simulink model "lab2sim"  (R2020a)
settings: Solver=VariableStepAuto  StartTime=0.0  StopTime=60  RelTol=1e-6
settings Model: Creator=ariana  LastModifiedBy=ariana

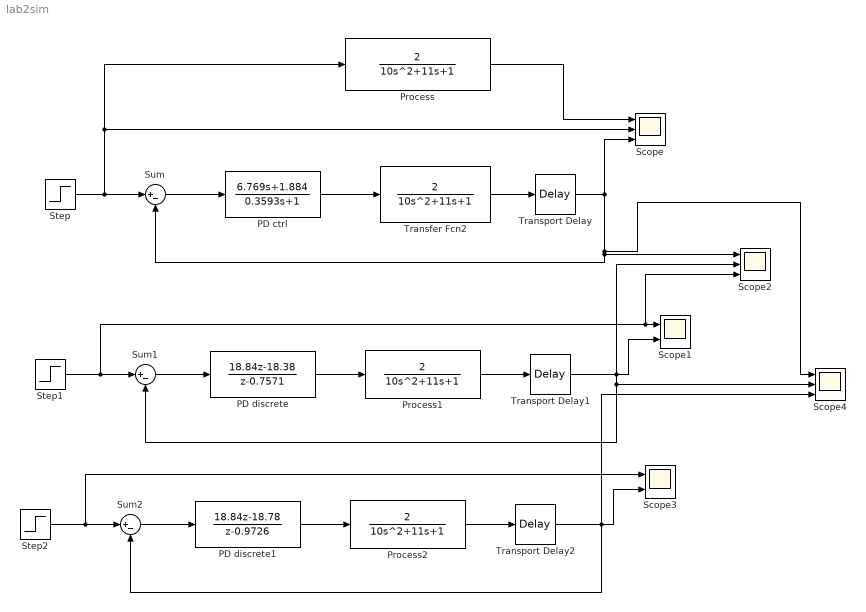
== system lab2sim ==
  " Process" : TransferFcn  Numerator=[2]  Denominator=[10 11 1]
  " Process1" : TransferFcn  Numerator=[2]  Denominator=[10 11 1]
  " Process2" : TransferFcn  Numerator=[2]  Denominator=[10 11 1]
  PD ctrl : TransferFcn  Numerator=[6.769 1.884]  Denominator=[0.3593 1]
  PD discrete : DiscreteTransferFcn  Numerator=[18.84 -18.38]  Denominator=[1 -0.7571]  SampleTime=0.1
  PD discrete1 : DiscreteTransferFcn  Numerator=[18.84 -18.78]  Denominator=[1 -0.9726]  SampleTime=0.01
  Scope : Scope  NumInputPorts=3
  Scope1 : Scope  NumInputPorts=2
  Scope2 : Scope  NumInputPorts=3
  Scope3 : Scope  NumInputPorts=2
  Scope4 : Scope  NumInputPorts=3
  Step : Step  Time=0  SampleTime=0
  Step1 : Step  Time=0  SampleTime=0
  Step2 : Step  Time=0  SampleTime=0
  Sum : Sum  Inputs=|+-
  Sum1 : Sum  Inputs=|+-
  Sum2 : Sum  Inputs=|+-
  Transfer Fcn2 : TransferFcn  Numerator=[2]  Denominator=[10 11 1]
  Transport Delay : TransportDelay
  Transport Delay1 : TransportDelay
  Transport Delay2 : TransportDelay
  wires:
  Step/1 -> " Process"/1, Scope/2, Sum/1
  Sum/1 -> PD ctrl/1
  PD ctrl/1 -> Transfer Fcn2/1
  Transfer Fcn2/1 -> Transport Delay/1
  Transport Delay/1 -> Scope4/1, Sum/2, Scope2/1, Scope/3
  " Process"/1 -> Scope/1
  PD discrete/1 -> " Process1"/1
  Sum1/1 -> PD discrete/1
  Step1/1 -> Scope2/3, Scope1/1, Sum1/1
  " Process1"/1 -> Transport Delay1/1
  Transport Delay1/1 -> Scope2/2, Scope4/2, Sum1/2, Scope1/2
  Sum2/1 -> PD discrete1/1
  " Process2"/1 -> Transport Delay2/1
  Transport Delay2/1 -> Scope4/3, Sum2/2, Scope3/2
  Step2/1 -> Scope3/1, Sum2/1
  PD discrete1/1 -> " Process2"/1
